simulink model "Longitudinal_Real"  (R2024b)
settings: Solver=VariableStepAuto  StartTime=0.0  StopTime=720  RelTol=1e-3
undefined symbols (not defined in the file): Kd_3, Ki_2, Ki_3, Ki_4, Ki_5, Kp_1, Kp_2, Kp_3, Kp_4, Kp_5
libraries: simulink x18, slpidlib x5
settings Model: Creator=GH-X-ST  LastModifiedBy=GH-X-ST

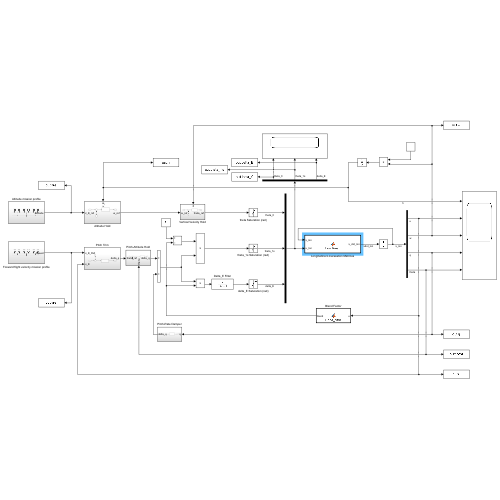
[thumbnail: Simulink's stored preview of the top-level diagram]
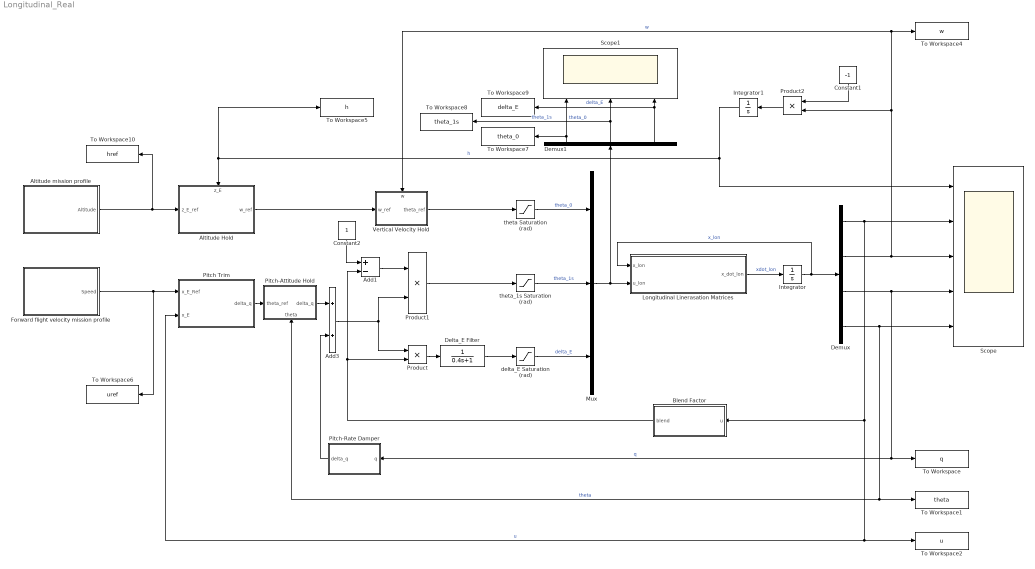
== system Longitudinal_Real ==
  Add1 : Sum  Inputs=+-
  Add3 : Sum
  Altitude Hold : Subsystem
      settings: PortSchema="{\"entries\":[{\"content\":{\"sides\":[{\"content\":{\"connectorIds\":[\"In1\"]},\"type\":\"ConnectorPlacement.EquallySpacedRectSide\",\"uuid\":\"786fe27b-9d32-4a4b-ba58-745251b51298\"},{\"content\":{\"connectorIds\":[\"Out1\"],\"side\":\"RIGHT\"},\"type\":\"ConnectorPlacement.EquallySpacedRectSide\",\"uuid\":\"c3e63844-28f7-4108-b9b9-8f5ae49ef2b7\"},{\"content\":{\"connectorIds\":[\"In2\"],\"side\":\"TOP\"},\"type\":\"ConnectorPlacement.EquallySpacedRectSide\",\"uuid\":\"709e7f88-d3c1-4cf0-9a6f-fe71781ed8e6\"}]},\"type\":\"ConnectorPlacement.EquallySpacedConnector\",\"uuid\":\"916bac8a-d735-4a54-bfae-f4eae304bdce\"}],\"packageUris\":[\"http://schema.mathworks.com/mf0/Connector/R2020b\"],\"version\":\"1.0\"}"
  Altitude mission profile : Subsystem
  Blend Factor : MATLAB Function  TreatAsAtomicUnit=on
  Constant1 : Constant  Value=-1
  Constant2 : Constant
  Delta_E Filter : TransferFcn  Denominator=[0.4 1]
  Demux : Demux
  Demux1 : Demux  Outputs=3
  Forward flight velocity mission profile : Subsystem
  Integrator : Integrator  InitialCondition=[0.000001; 0; 0; 0]
  Integrator1 : Integrator  InitialCondition=135  ContinuousStateAttributes='h'
  Longitudinal Linerasation Matrices : MATLAB Function  TreatAsAtomicUnit=on
  Mux : Mux  Inputs=3
  Pitch Trim : Subsystem
  Pitch-Attitude Hold : Subsystem
      settings: PortSchema="{\"entries\":[{\"content\":{\"sides\":[{\"content\":{\"connectorIds\":[\"In1\"]},\"type\":\"ConnectorPlacement.EquallySpacedRectSide\",\"uuid\":\"6ee333b9-9b69-42fd-975a-4580f9624540\"},{\"content\":{\"connectorIds\":[\"Out1\"],\"side\":\"RIGHT\"},\"type\":\"ConnectorPlacement.EquallySpacedRectSide\",\"uuid\":\"6a43d978-a0a5-4636-bfdb-b097e996a039\"},{\"content\":{\"side\":\"TOP\"},\"type\":\"ConnectorPlacement.EquallySpacedRectSide\",\"uuid\":\"00f937d1-ecc9-42d4-adf8-d8f1b79c75a6\"},{\"content\":{\"connectorIds\":[\"In2\"],\"side\":\"BOTTOM\"},\"type\":\"ConnectorPlacement.EquallySpacedRectSide\",\"uuid\":\"809403f9-594f-4491-8a7d-ee0f8643f57e\"}]},\"type\":\"ConnectorPlacement.EquallySpacedConnector\",\"uuid\":\"362aafbc-ebc0-4bb3-8c4e-be284a8bc83f\"}],\"packageUris\":[\"http://schema.mathworks.com/mf0/Connector/R2020b\"],\"version\":\"1.0\"}"
  Pitch-Rate Damper : Subsystem
  Product : Product
  Product1 : Product
  Product2 : Product
  Scope : Scope  NumInputPorts=5
  Scope1 : Scope  NumInputPorts=3
  To Workspace : ToWorkspace  VariableName=q  SaveFormat=Timeseries  SampleTime=-1
  To Workspace1 : ToWorkspace  VariableName=theta  SaveFormat=Timeseries  SampleTime=-1
  To Workspace10 : ToWorkspace  VariableName=href  SaveFormat=Timeseries  SampleTime=-1
  To Workspace2 : ToWorkspace  VariableName=u  SaveFormat=Timeseries  SampleTime=-1
  To Workspace4 : ToWorkspace  VariableName=w  SaveFormat=Timeseries  SampleTime=-1
  To Workspace5 : ToWorkspace  VariableName=h  SaveFormat=Timeseries  SampleTime=-1
  To Workspace6 : ToWorkspace  VariableName=uref  SaveFormat=Timeseries  SampleTime=-1
  To Workspace7 : ToWorkspace  VariableName=theta_0  SaveFormat=Timeseries  SampleTime=-1
  To Workspace8 : ToWorkspace  VariableName=theta_1s  SaveFormat=Timeseries  SampleTime=-1
  To Workspace9 : ToWorkspace  VariableName=delta_E  SaveFormat=Timeseries  SampleTime=-1
  Vertical Velocity Hold : Subsystem
      settings: PortSchema="{\"entries\":[{\"content\":{\"sides\":[{\"content\":{\"connectorIds\":[\"In1\"]},\"type\":\"ConnectorPlacement.EquallySpacedRectSide\",\"uuid\":\"6ee333b9-9b69-42fd-975a-4580f9624540\"},{\"content\":{\"connectorIds\":[\"Out1\"],\"side\":\"RIGHT\"},\"type\":\"ConnectorPlacement.EquallySpacedRectSide\",\"uuid\":\"6a43d978-a0a5-4636-bfdb-b097e996a039\"},{\"content\":{\"connectorIds\":[\"In2\"],\"side\":\"TOP\"},\"type\":\"ConnectorPlacement.EquallySpacedRectSide\",\"uuid\":\"00f937d1-ecc9-42d4-adf8-d8f1b79c75a6\"},{\"content\":{\"side\":\"BOTTOM\"},\"type\":\"ConnectorPlacement.EquallySpacedRectSide\",\"uuid\":\"64d125d6-056c-4640-9df5-5340aaf5f7d1\"}]},\"type\":\"ConnectorPlacement.EquallySpacedConnector\",\"uuid\":\"362aafbc-ebc0-4bb3-8c4e-be284a8bc83f\"}],\"packageUris\":[\"http://schema.mathworks.com/mf0/Connector/R2020b\"],\"version\":\"1.0\"}"
  delta_E Saturation (rad) : Saturate  UpperLimit=deg2rad(11)  LowerLimit=deg2rad(-11)
  theta Saturation (rad) : Saturate  UpperLimit=deg2rad(+20)  LowerLimit=deg2rad(-6)
  theta_1s Saturation (rad) : Saturate  UpperLimit=deg2rad(6)  LowerLimit=deg2rad(-6)
  wires:
  Longitudinal Linerasation Matrices/1(x_dot_lon) -> Integrator/1  "xdot_lon"
  Integrator/1 -> Longitudinal Linerasation Matrices/1(x_lon), Demux/1  "x_lon"
  Demux/1 -> Scope/2, Blend Factor/1(u), To Workspace2/1, Pitch Trim/2(x_E)  "u"
  Demux/2 -> Vertical Velocity Hold/2(w), To Workspace4/1, Product2/2, Scope/3  "w"
  Demux/3 -> Scope/4, To Workspace/1, Pitch-Rate Damper/1(q)  "q"
  Demux/4 -> Scope/5, To Workspace1/1, Pitch-Attitude Hold/2(theta)  "theta"
  Blend Factor/1(blend) -> Add1/2, Product/2
  Pitch-Attitude Hold/1(delta_q) -> Add3/1
  Constant2/1 -> Add1/1
  Add1/1 -> Product1/1
  Mux/1 -> Demux1/1, Longitudinal Linerasation Matrices/2(u_lon)
  Demux1/3 -> To Workspace9/1, Scope1/3  "delta_E"
  Demux1/2 -> Scope1/2, To Workspace8/1  "theta_1s"
  Demux1/1 -> Scope1/1, To Workspace7/1  "theta_0"
  Product/1 -> Delta_E Filter/1
  Pitch-Rate Damper/1(delta_q) -> Add3/2
  Constant1/1 -> Product2/1
  Product2/1 -> Integrator1/1
  Integrator1/1 -> Scope/1, Altitude Hold/2(z_E), To Workspace5/1  "h"
  Altitude Hold/1(w_ref) -> Vertical Velocity Hold/1(w_ref)
  Add3/1 -> Product1/2, Product/1
  Pitch Trim/1(delta_q) -> Pitch-Attitude Hold/1(theta_ref)
  Delta_E Filter/1 -> delta_E Saturation (rad)/1
  delta_E Saturation (rad)/1 -> Mux/3  "delta_E"
  theta_1s Saturation (rad)/1 -> Mux/2  "theta_1s"
  Product1/1 -> theta_1s Saturation (rad)/1
  Vertical Velocity Hold/1(theta_ref) -> theta Saturation (rad)/1
  theta Saturation (rad)/1 -> Mux/1  "theta_0"
  Altitude mission profile/1(Altitude) -> To Workspace10/1, Altitude Hold/1(z_E_ref)
  Forward flight velocity mission profile/1(Speed) -> To Workspace6/1, Pitch Trim/1(x_E_Ref)

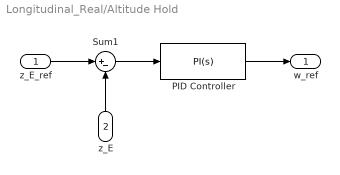
== system Longitudinal_Real/Altitude Hold ==
  z_E_ref : Inport
  z_E : Inport  Port=2
  PID Controller : slpidlib/PID Controller  Controller=PI  Form=Parallel  TimeDomain=Continuous-time  UseExternalTs=off  SampleTime=-1  IntegratorMethod=Forward Euler  FilterMethod=Forward Euler  ControllerParametersSource=internal  P=Kp_5  I=Ki_5  UseKiTs=off  D=0.005  UseExternalDerivativeSource=off  N=100  UseFilter=on  TunerSelectOption=Transfer Function Based (PID Tuner App)  InitialConditionSource=internal  InitialConditionForIntegrator=0  InitialConditionForFilter=0  DifferentiatorICPrevScaledInput=0  ExternalReset=none  TrackingMode=off  Kt=1  LimitOutput=on  SatLimitsSource=internal  UpperSaturationLimit=1  LowerSaturationLimit=-1  LinearizeAsGain=on  AntiWindupMode=none  Kb=1  LimitIntegrator=off  UpperIntegratorSaturationLimit=inf  LowerIntegratorSaturationLimit=-inf  POutMin=[]  POutMax=[]  IOutMin=[]  IOutMax=[]  DOutMin=[]  DOutMax=[]  NOutMin=[]  NOutMax=[]  SumOutMin=[]  SumOutMax=[]  SaturationOutMin=[]  SaturationOutMax=[]  PParamMin=[]  PParamMax=[]  IParamMin=[]  IParamMax=[]  DParamMin=[]  DParamMax=[]  NParamMin=[]  NParamMax=[]  KbParamMin=[]  KbParamMax=[]  KtParamMin=[]  KtParamMax=[]  KbOutMin=[]  KbOutMax=[]  KtOutMin=[]  KtOutMax=[]  IntegratorOutMin=[]  IntegratorOutMax=[]  FilterOutMin=[]  FilterOutMax=[]  SumI1OutMin=[]  SumI1OutMax=[]  SumI2OutMin=[]  SumI2OutMax=[]  SumI3OutMin=[]  SumI3OutMax=[]  SumI4OutMin=[]  SumI4OutMax=[]  SumDOutMin=[]  SumDOutMax=[]  DifferentiatorOutMin=[]  DifferentiatorOutMax=[]  FilterDiffOutCoefMin=[]  FilterDiffOutCoefMax=[]  ReciprocalOutMin=[]  ReciprocalOutMax=[]  SumDenOutMin=[]  SumDenOutMax=[]  SumNumOutMin=[]  SumNumOutMax=[]  DivideOutMin=[]  DivideOutMax=[]  UdiffTsProdOutMin=[]  UdiffTsProdOutMax=[]  NTsProdOutMin=[]  NTsProdOutMax=[]  UintegralTsProdOutMin=[]  UintegralTsProdOutMax=[]  UngainTsProdOutMin=[]  UngainTsProdOutMax=[]  ClampingZeroOutDataTypeStr=Inherit: Inherit via back propagation  ClampingZeroOutMin=[]  ClampingZeroOutMax=[]  FilterDenConstantOutDataTypeStr=Inherit: Inherit via back propagation  FilterDenConstantOutMin=[]  FilterDenConstantOutMax=[]  PCopyOutDataTypeStr=Inherit: Inherit via back propagation  PCopyOutMin=[]  PCopyOutMax=[]  NCopyOutDataTypeStr=Inherit: Inherit via back propagation  NCopyOutMin=[]  NCopyOutMax=[]  IntegratorContinuousStateAttributes=''  IntegratorStateMustResolveToSignalObject=off  IntegratorRTWStateStorageClass=Auto  FilterContinuousStateAttributes=''  FilterStateMustResolveToSignalObject=off  FilterRTWStateStorageClass=Auto  ParallelPVariant=InternalParameters  IdealPVariant=Disabled  IVariant=InternalParameters  DVariant=Disabled  IntegratorVariant=Continuous  SatVariant=Enabled  AWVariant=Passthrough  PCopyVariant=Disabled  TRVariant=Disabled  FdbkBlocksVariant=Forward  IdealPFdbkVariant=Disabled  SatFdbkVariant=Disabled  DerivativeFilterVariant=Disabled  NVariant=Disabled  NCopyVariant=Disabled_SignalSpec  FilterICVariant=Disabled  IntegratorICVariant=InternalICs  ExternalResetVariant=Disabled  TRSumVariant=Passthrough  SumFdbkVariant=Disabled  SumVariant=Sum_PI  TsampFilterVariant=InternalTs  TsampNgainVariant=Passthrough  TsampIntegralVariant=Disabled_SignalSpec  ExternalSaturationOutDataTypeStr=Inherit: Same as second input  DerivativeSourceVariant=Disabled  PreIntVariant=InternalPreInt
  Sum1 : Sum  Inputs=|+-
  w_ref : Outport
  wires:
  PID Controller/1 -> w_ref/1
  Sum1/1 -> PID Controller/1
  z_E_ref/1 -> Sum1/1
  z_E/1 -> Sum1/2

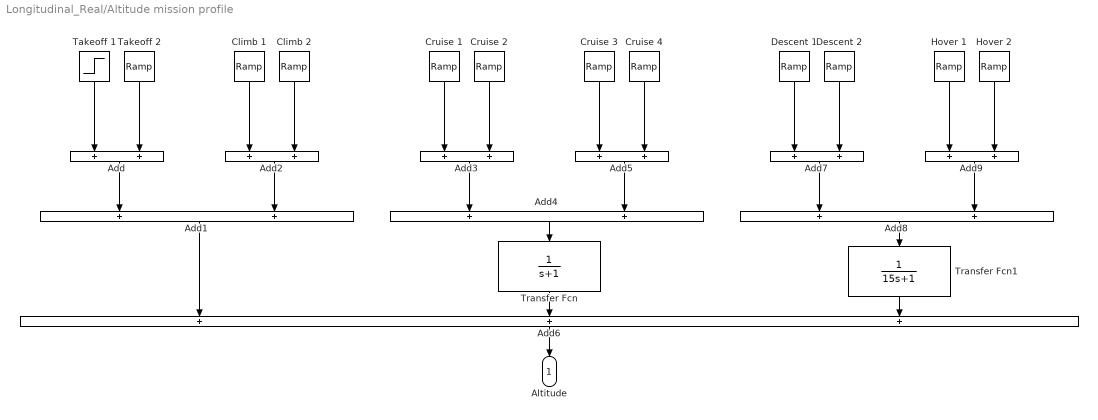
== system Longitudinal_Real/Altitude mission profile ==
  Add{,1..5,7..9} (9 alike) : Sum
  Add6 : Sum  Inputs=+++
  Climb 1 : simulink/Sources/Ramp  slope=0.4  start=50  InitialOutput=0
  Climb 2 : simulink/Sources/Ramp  slope=-0.4  start=100  InitialOutput=0
  Cruise 1 : simulink/Sources/Ramp  slope=0.1  start=100  InitialOutput=0
  Cruise 2 : simulink/Sources/Ramp  slope=-0.1  start=200  InitialOutput=0
  Cruise 3 : simulink/Sources/Ramp  slope=0  start=200  InitialOutput=0
  Cruise 4 : simulink/Sources/Ramp  slope=0  start=350  InitialOutput=0
  Descent 1 : simulink/Sources/Ramp  slope=-12/70  start=350  InitialOutput=0
  Descent 2 : simulink/Sources/Ramp  slope=12/70  start=475  InitialOutput=0
  Hover 1 : simulink/Sources/Ramp  slope=0  start=475  InitialOutput=0
  Hover 2 : simulink/Sources/Ramp  slope=0  start=600  InitialOutput=0
  Takeoff 1 : Step  Time=0  Before=135  After=150  SampleTime=0
  Takeoff 2 : simulink/Sources/Ramp  slope=0  start=50  InitialOutput=0
  Transfer Fcn : TransferFcn  Denominator=[1 1]
  Transfer Fcn1 : TransferFcn  Denominator=[15 1]
  Altitude : Outport
  wires:
  Add1/1 -> Add6/1
  Climb 2/1 -> Add2/2
  Add4/1 -> Transfer Fcn/1
  Climb 1/1 -> Add2/1
  Hover 1/1 -> Add9/1
  Add7/1 -> Add8/1
  Descent 1/1 -> Add7/1
  Add9/1 -> Add8/2
  Hover 2/1 -> Add9/2
  Add8/1 -> Transfer Fcn1/1
  Add2/1 -> Add1/2
  Add3/1 -> Add4/1
  Add5/1 -> Add4/2
  Cruise 2/1 -> Add3/2
  Cruise 4/1 -> Add5/2
  Cruise 1/1 -> Add3/1
  Cruise 3/1 -> Add5/1
  Descent 2/1 -> Add7/2
  Takeoff 2/1 -> Add/2
  Takeoff 1/1 -> Add/1
  Add/1 -> Add1/1
  Add6/1 -> Altitude/1
  Transfer Fcn/1 -> Add6/2
  Transfer Fcn1/1 -> Add6/3

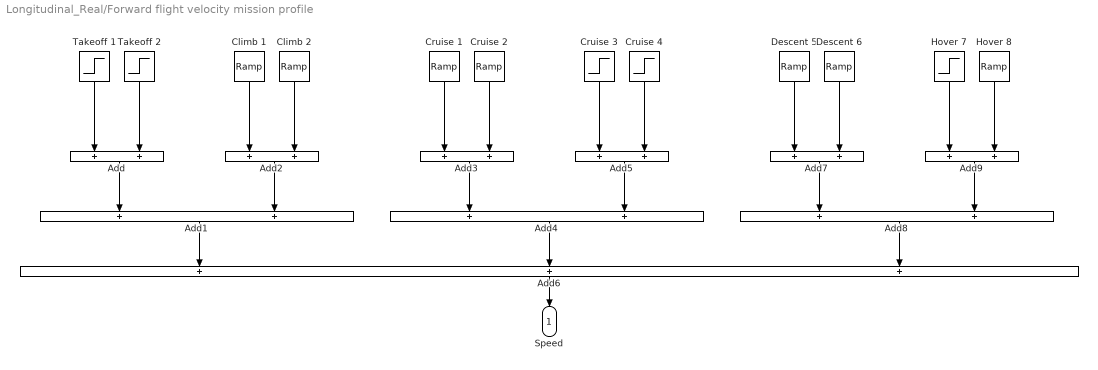
== system Longitudinal_Real/Forward flight velocity mission profile ==
  Add{,1..5,7..9} (9 alike) : Sum
  Add6 : Sum  Inputs=+++
  Climb 1 : simulink/Sources/Ramp  slope=0.4  start=50  InitialOutput=0
  Climb 2 : simulink/Sources/Ramp  slope=-0.4  start=100  InitialOutput=0
  Cruise 1 : simulink/Sources/Ramp  slope=0  start=100  InitialOutput=0
  Cruise 2 : simulink/Sources/Ramp  slope=0  start=200  InitialOutput=0
  Cruise 3 : Step  Time=200  After=22  SampleTime=0
  Cruise 4 : Step  Time=350  After=-37  SampleTime=0
  Descent 5 : simulink/Sources/Ramp  slope=0  start=350  InitialOutput=0
  Descent 6 : simulink/Sources/Ramp  slope=0  start=475  InitialOutput=0
  Hover 7 : Step  Time=475  After=-35  SampleTime=0
  Hover 8 : simulink/Sources/Ramp  slope=0  start=600  InitialOutput=0
  Takeoff 1 : Step  Time=0  After=0  SampleTime=0
  Takeoff 2 : Step  Time=50  After=30  SampleTime=0
  Speed : Outport
  wires:
  Add6/1 -> Speed/1
  Add1/1 -> Add6/1
  Climb 2/1 -> Add2/2
  Add4/1 -> Add6/2
  Climb 1/1 -> Add2/1
  Add7/1 -> Add8/1
  Descent 5/1 -> Add7/1
  Add9/1 -> Add8/2
  Descent 6/1 -> Add7/2
  Hover 8/1 -> Add9/2
  Add8/1 -> Add6/3
  Add2/1 -> Add1/2
  Add3/1 -> Add4/1
  Add5/1 -> Add4/2
  Cruise 1/1 -> Add3/1
  Cruise 4/1 -> Add5/2
  Add/1 -> Add1/1
  Hover 7/1 -> Add9/1
  Takeoff 1/1 -> Add/1
  Takeoff 2/1 -> Add/2
  Cruise 3/1 -> Add5/1
  Cruise 2/1 -> Add3/2

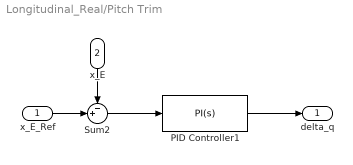
== system Longitudinal_Real/Pitch Trim ==
  x_E_Ref : Inport
  x_E : Inport  Port=2
  PID Controller1 : slpidlib/PID Controller  Controller=PI  Form=Parallel  TimeDomain=Continuous-time  UseExternalTs=off  SampleTime=-1  IntegratorMethod=Forward Euler  FilterMethod=Forward Euler  ControllerParametersSource=internal  P=Kp_3  I=Ki_3  UseKiTs=off  D=Kd_3  UseExternalDerivativeSource=off  N=100  UseFilter=on  TunerSelectOption=Transfer Function Based (PID Tuner App)  InitialConditionSource=internal  InitialConditionForIntegrator=0  InitialConditionForFilter=0  DifferentiatorICPrevScaledInput=0  ExternalReset=none  TrackingMode=off  Kt=1  LimitOutput=on  SatLimitsSource=internal  UpperSaturationLimit=1  LowerSaturationLimit=-1  LinearizeAsGain=on  AntiWindupMode=none  Kb=1  LimitIntegrator=off  UpperIntegratorSaturationLimit=inf  LowerIntegratorSaturationLimit=-inf  POutMin=[]  POutMax=[]  IOutMin=[]  IOutMax=[]  DOutMin=[]  DOutMax=[]  NOutMin=[]  NOutMax=[]  SumOutMin=[]  SumOutMax=[]  SaturationOutMin=[]  SaturationOutMax=[]  PParamMin=[]  PParamMax=[]  IParamMin=[]  IParamMax=[]  DParamMin=[]  DParamMax=[]  NParamMin=[]  NParamMax=[]  KbParamMin=[]  KbParamMax=[]  KtParamMin=[]  KtParamMax=[]  KbOutMin=[]  KbOutMax=[]  KtOutMin=[]  KtOutMax=[]  IntegratorOutMin=[]  IntegratorOutMax=[]  FilterOutMin=[]  FilterOutMax=[]  SumI1OutMin=[]  SumI1OutMax=[]  SumI2OutMin=[]  SumI2OutMax=[]  SumI3OutMin=[]  SumI3OutMax=[]  SumI4OutMin=[]  SumI4OutMax=[]  SumDOutMin=[]  SumDOutMax=[]  DifferentiatorOutMin=[]  DifferentiatorOutMax=[]  FilterDiffOutCoefMin=[]  FilterDiffOutCoefMax=[]  ReciprocalOutMin=[]  ReciprocalOutMax=[]  SumDenOutMin=[]  SumDenOutMax=[]  SumNumOutMin=[]  SumNumOutMax=[]  DivideOutMin=[]  DivideOutMax=[]  UdiffTsProdOutMin=[]  UdiffTsProdOutMax=[]  NTsProdOutMin=[]  NTsProdOutMax=[]  UintegralTsProdOutMin=[]  UintegralTsProdOutMax=[]  UngainTsProdOutMin=[]  UngainTsProdOutMax=[]  ClampingZeroOutDataTypeStr=Inherit: Inherit via back propagation  ClampingZeroOutMin=[]  ClampingZeroOutMax=[]  FilterDenConstantOutDataTypeStr=Inherit: Inherit via back propagation  FilterDenConstantOutMin=[]  FilterDenConstantOutMax=[]  PCopyOutDataTypeStr=Inherit: Inherit via back propagation  PCopyOutMin=[]  PCopyOutMax=[]  NCopyOutDataTypeStr=Inherit: Inherit via back propagation  NCopyOutMin=[]  NCopyOutMax=[]  IntegratorContinuousStateAttributes=''  IntegratorStateMustResolveToSignalObject=off  IntegratorRTWStateStorageClass=Auto  FilterContinuousStateAttributes=''  FilterStateMustResolveToSignalObject=off  FilterRTWStateStorageClass=Auto  ParallelPVariant=InternalParameters  IdealPVariant=Disabled  IVariant=InternalParameters  DVariant=Disabled  IntegratorVariant=Continuous  SatVariant=Enabled  AWVariant=Passthrough  PCopyVariant=Disabled  TRVariant=Disabled  FdbkBlocksVariant=Forward  IdealPFdbkVariant=Disabled  SatFdbkVariant=Disabled  DerivativeFilterVariant=Disabled  NVariant=Disabled  NCopyVariant=Disabled_SignalSpec  FilterICVariant=Disabled  IntegratorICVariant=InternalICs  ExternalResetVariant=Disabled  TRSumVariant=Passthrough  SumFdbkVariant=Disabled  SumVariant=Sum_PI  TsampFilterVariant=InternalTs  TsampNgainVariant=Passthrough  TsampIntegralVariant=Disabled_SignalSpec  ExternalSaturationOutDataTypeStr=Inherit: Same as second input  DerivativeSourceVariant=Disabled  PreIntVariant=InternalPreInt
  Sum2 : Sum  Inputs=-+|
  delta_q : Outport
  wires:
  x_E/1 -> Sum2/1
  x_E_Ref/1 -> Sum2/2
  PID Controller1/1 -> delta_q/1
  Sum2/1 -> PID Controller1/1

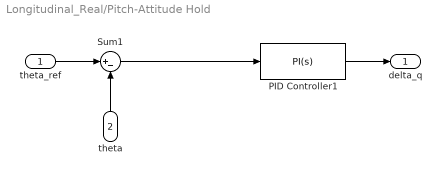
== system Longitudinal_Real/Pitch-Attitude Hold ==
  theta_ref : Inport
  theta : Inport  Port=2
  PID Controller1 : slpidlib/PID Controller  Controller=PI  Form=Parallel  TimeDomain=Continuous-time  UseExternalTs=off  SampleTime=-1  IntegratorMethod=Forward Euler  FilterMethod=Forward Euler  ControllerParametersSource=internal  P=Kp_2  I=Ki_2  UseKiTs=off  D=0.005  UseExternalDerivativeSource=on  N=100  UseFilter=on  TunerSelectOption=Transfer Function Based (PID Tuner App)  InitialConditionSource=internal  InitialConditionForIntegrator=0  InitialConditionForFilter=0  DifferentiatorICPrevScaledInput=0  ExternalReset=none  TrackingMode=off  Kt=1  LimitOutput=on  SatLimitsSource=internal  UpperSaturationLimit=1  LowerSaturationLimit=-1  LinearizeAsGain=on  AntiWindupMode=none  Kb=1  LimitIntegrator=off  UpperIntegratorSaturationLimit=inf  LowerIntegratorSaturationLimit=-inf  POutMin=[]  POutMax=[]  IOutMin=[]  IOutMax=[]  DOutMin=[]  DOutMax=[]  NOutMin=[]  NOutMax=[]  SumOutMin=[]  SumOutMax=[]  SaturationOutMin=[]  SaturationOutMax=[]  PParamMin=[]  PParamMax=[]  IParamMin=[]  IParamMax=[]  DParamMin=[]  DParamMax=[]  NParamMin=[]  NParamMax=[]  KbParamMin=[]  KbParamMax=[]  KtParamMin=[]  KtParamMax=[]  KbOutMin=[]  KbOutMax=[]  KtOutMin=[]  KtOutMax=[]  IntegratorOutMin=[]  IntegratorOutMax=[]  FilterOutMin=[]  FilterOutMax=[]  SumI1OutMin=[]  SumI1OutMax=[]  SumI2OutMin=[]  SumI2OutMax=[]  SumI3OutMin=[]  SumI3OutMax=[]  SumI4OutMin=[]  SumI4OutMax=[]  SumDOutMin=[]  SumDOutMax=[]  DifferentiatorOutMin=[]  DifferentiatorOutMax=[]  FilterDiffOutCoefMin=[]  FilterDiffOutCoefMax=[]  ReciprocalOutMin=[]  ReciprocalOutMax=[]  SumDenOutMin=[]  SumDenOutMax=[]  SumNumOutMin=[]  SumNumOutMax=[]  DivideOutMin=[]  DivideOutMax=[]  UdiffTsProdOutMin=[]  UdiffTsProdOutMax=[]  NTsProdOutMin=[]  NTsProdOutMax=[]  UintegralTsProdOutMin=[]  UintegralTsProdOutMax=[]  UngainTsProdOutMin=[]  UngainTsProdOutMax=[]  ClampingZeroOutDataTypeStr=Inherit: Inherit via back propagation  ClampingZeroOutMin=[]  ClampingZeroOutMax=[]  FilterDenConstantOutDataTypeStr=Inherit: Inherit via back propagation  FilterDenConstantOutMin=[]  FilterDenConstantOutMax=[]  PCopyOutDataTypeStr=Inherit: Inherit via back propagation  PCopyOutMin=[]  PCopyOutMax=[]  NCopyOutDataTypeStr=Inherit: Inherit via back propagation  NCopyOutMin=[]  NCopyOutMax=[]  IntegratorContinuousStateAttributes=''  IntegratorStateMustResolveToSignalObject=off  IntegratorRTWStateStorageClass=Auto  FilterContinuousStateAttributes=''  FilterStateMustResolveToSignalObject=off  FilterRTWStateStorageClass=Auto  ParallelPVariant=InternalParameters  IdealPVariant=Disabled  IVariant=InternalParameters  DVariant=Disabled  IntegratorVariant=Continuous  SatVariant=Enabled  AWVariant=Passthrough  PCopyVariant=Disabled  TRVariant=Disabled  FdbkBlocksVariant=Forward  IdealPFdbkVariant=Disabled  SatFdbkVariant=Disabled  DerivativeFilterVariant=Disabled  NVariant=Passthrough  NCopyVariant=Disabled_SignalSpec  FilterICVariant=Disabled  IntegratorICVariant=InternalICs  ExternalResetVariant=Disabled  TRSumVariant=Passthrough  SumFdbkVariant=Disabled  SumVariant=Sum_PI  TsampFilterVariant=InternalTs  TsampNgainVariant=Passthrough  TsampIntegralVariant=Disabled_SignalSpec  ExternalSaturationOutDataTypeStr=Inherit: Same as second input  DerivativeSourceVariant=Disabled  PreIntVariant=InternalPreInt
  Sum1 : Sum  Inputs=|+-
  delta_q : Outport
  wires:
  PID Controller1/1 -> delta_q/1
  theta_ref/1 -> Sum1/1
  theta/1 -> Sum1/2
  Sum1/1 -> PID Controller1/1

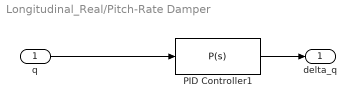
== system Longitudinal_Real/Pitch-Rate Damper ==
  q : Inport
  PID Controller1 : slpidlib/PID Controller  Controller=P  Form=Parallel  TimeDomain=Continuous-time  UseExternalTs=off  SampleTime=-1  IntegratorMethod=Forward Euler  FilterMethod=Forward Euler  ControllerParametersSource=internal  P=Kp_1  I=0.005  UseKiTs=off  D=0.005  UseExternalDerivativeSource=on  N=100  UseFilter=on  TunerSelectOption=Transfer Function Based (PID Tuner App)  InitialConditionSource=internal  InitialConditionForIntegrator=0  InitialConditionForFilter=0  DifferentiatorICPrevScaledInput=0  ExternalReset=none  TrackingMode=off  Kt=1  LimitOutput=on  SatLimitsSource=internal  UpperSaturationLimit=1  LowerSaturationLimit=-1  LinearizeAsGain=on  AntiWindupMode=none  Kb=1  LimitIntegrator=off  UpperIntegratorSaturationLimit=inf  LowerIntegratorSaturationLimit=-inf  POutMin=[]  POutMax=[]  IOutMin=[]  IOutMax=[]  DOutMin=[]  DOutMax=[]  NOutMin=[]  NOutMax=[]  SumOutMin=[]  SumOutMax=[]  SaturationOutMin=[]  SaturationOutMax=[]  PParamMin=[]  PParamMax=[]  IParamMin=[]  IParamMax=[]  DParamMin=[]  DParamMax=[]  NParamMin=[]  NParamMax=[]  KbParamMin=[]  KbParamMax=[]  KtParamMin=[]  KtParamMax=[]  KbOutMin=[]  KbOutMax=[]  KtOutMin=[]  KtOutMax=[]  IntegratorOutMin=[]  IntegratorOutMax=[]  FilterOutMin=[]  FilterOutMax=[]  SumI1OutMin=[]  SumI1OutMax=[]  SumI2OutMin=[]  SumI2OutMax=[]  SumI3OutMin=[]  SumI3OutMax=[]  SumI4OutMin=[]  SumI4OutMax=[]  SumDOutMin=[]  SumDOutMax=[]  DifferentiatorOutMin=[]  DifferentiatorOutMax=[]  FilterDiffOutCoefMin=[]  FilterDiffOutCoefMax=[]  ReciprocalOutMin=[]  ReciprocalOutMax=[]  SumDenOutMin=[]  SumDenOutMax=[]  SumNumOutMin=[]  SumNumOutMax=[]  DivideOutMin=[]  DivideOutMax=[]  UdiffTsProdOutMin=[]  UdiffTsProdOutMax=[]  NTsProdOutMin=[]  NTsProdOutMax=[]  UintegralTsProdOutMin=[]  UintegralTsProdOutMax=[]  UngainTsProdOutMin=[]  UngainTsProdOutMax=[]  ClampingZeroOutDataTypeStr=Inherit: Inherit via back propagation  ClampingZeroOutMin=[]  ClampingZeroOutMax=[]  FilterDenConstantOutDataTypeStr=Inherit: Inherit via back propagation  FilterDenConstantOutMin=[]  FilterDenConstantOutMax=[]  PCopyOutDataTypeStr=Inherit: Inherit via back propagation  PCopyOutMin=[]  PCopyOutMax=[]  NCopyOutDataTypeStr=Inherit: Inherit via back propagation  NCopyOutMin=[]  NCopyOutMax=[]  IntegratorContinuousStateAttributes=''  IntegratorStateMustResolveToSignalObject=off  IntegratorRTWStateStorageClass=Auto  FilterContinuousStateAttributes=''  FilterStateMustResolveToSignalObject=off  FilterRTWStateStorageClass=Auto  ParallelPVariant=InternalParameters  IdealPVariant=Disabled  IVariant=Disabled  DVariant=Disabled  IntegratorVariant=Disabled  SatVariant=Enabled  AWVariant=Disabled  PCopyVariant=Disabled  TRVariant=Disabled  FdbkBlocksVariant=Forward  IdealPFdbkVariant=Disabled  SatFdbkVariant=Disabled  DerivativeFilterVariant=Disabled  NVariant=Passthrough  NCopyVariant=Disabled_SignalSpec  FilterICVariant=Disabled  IntegratorICVariant=Disabled  ExternalResetVariant=Disabled  TRSumVariant=Passthrough  SumFdbkVariant=Disabled  SumVariant=Passthrough_P  TsampFilterVariant=InternalTs  TsampNgainVariant=Passthrough  TsampIntegralVariant=Disabled_SignalSpec  ExternalSaturationOutDataTypeStr=Inherit: Same as second input  DerivativeSourceVariant=Disabled  PreIntVariant=InternalPreInt
  delta_q : Outport
  wires:
  PID Controller1/1 -> delta_q/1
  q/1 -> PID Controller1/1

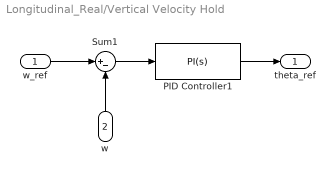
== system Longitudinal_Real/Vertical Velocity Hold ==
  w_ref : Inport
  w : Inport  Port=2
  PID Controller1 : slpidlib/PID Controller  Controller=PI  Form=Parallel  TimeDomain=Continuous-time  UseExternalTs=off  SampleTime=-1  IntegratorMethod=Forward Euler  FilterMethod=Forward Euler  ControllerParametersSource=internal  P=Kp_4  I=Ki_4  UseKiTs=off  D=0.005  UseExternalDerivativeSource=on  N=100  UseFilter=on  TunerSelectOption=Transfer Function Based (PID Tuner App)  InitialConditionSource=internal  InitialConditionForIntegrator=0  InitialConditionForFilter=0  DifferentiatorICPrevScaledInput=0  ExternalReset=none  TrackingMode=off  Kt=1  LimitOutput=on  SatLimitsSource=internal  UpperSaturationLimit=1  LowerSaturationLimit=-1  LinearizeAsGain=on  AntiWindupMode=none  Kb=1  LimitIntegrator=off  UpperIntegratorSaturationLimit=inf  LowerIntegratorSaturationLimit=-inf  POutMin=[]  POutMax=[]  IOutMin=[]  IOutMax=[]  DOutMin=[]  DOutMax=[]  NOutMin=[]  NOutMax=[]  SumOutMin=[]  SumOutMax=[]  SaturationOutMin=[]  SaturationOutMax=[]  PParamMin=[]  PParamMax=[]  IParamMin=[]  IParamMax=[]  DParamMin=[]  DParamMax=[]  NParamMin=[]  NParamMax=[]  KbParamMin=[]  KbParamMax=[]  KtParamMin=[]  KtParamMax=[]  KbOutMin=[]  KbOutMax=[]  KtOutMin=[]  KtOutMax=[]  IntegratorOutMin=[]  IntegratorOutMax=[]  FilterOutMin=[]  FilterOutMax=[]  SumI1OutMin=[]  SumI1OutMax=[]  SumI2OutMin=[]  SumI2OutMax=[]  SumI3OutMin=[]  SumI3OutMax=[]  SumI4OutMin=[]  SumI4OutMax=[]  SumDOutMin=[]  SumDOutMax=[]  DifferentiatorOutMin=[]  DifferentiatorOutMax=[]  FilterDiffOutCoefMin=[]  FilterDiffOutCoefMax=[]  ReciprocalOutMin=[]  ReciprocalOutMax=[]  SumDenOutMin=[]  SumDenOutMax=[]  SumNumOutMin=[]  SumNumOutMax=[]  DivideOutMin=[]  DivideOutMax=[]  UdiffTsProdOutMin=[]  UdiffTsProdOutMax=[]  NTsProdOutMin=[]  NTsProdOutMax=[]  UintegralTsProdOutMin=[]  UintegralTsProdOutMax=[]  UngainTsProdOutMin=[]  UngainTsProdOutMax=[]  ClampingZeroOutDataTypeStr=Inherit: Inherit via back propagation  ClampingZeroOutMin=[]  ClampingZeroOutMax=[]  FilterDenConstantOutDataTypeStr=Inherit: Inherit via back propagation  FilterDenConstantOutMin=[]  FilterDenConstantOutMax=[]  PCopyOutDataTypeStr=Inherit: Inherit via back propagation  PCopyOutMin=[]  PCopyOutMax=[]  NCopyOutDataTypeStr=Inherit: Inherit via back propagation  NCopyOutMin=[]  NCopyOutMax=[]  IntegratorContinuousStateAttributes=''  IntegratorStateMustResolveToSignalObject=off  IntegratorRTWStateStorageClass=Auto  FilterContinuousStateAttributes=''  FilterStateMustResolveToSignalObject=off  FilterRTWStateStorageClass=Auto  ParallelPVariant=InternalParameters  IdealPVariant=Disabled  IVariant=InternalParameters  DVariant=Disabled  IntegratorVariant=Continuous  SatVariant=Enabled  AWVariant=Passthrough  PCopyVariant=Disabled  TRVariant=Disabled  FdbkBlocksVariant=Forward  IdealPFdbkVariant=Disabled  SatFdbkVariant=Disabled  DerivativeFilterVariant=Disabled  NVariant=Passthrough  NCopyVariant=Disabled_SignalSpec  FilterICVariant=Disabled  IntegratorICVariant=InternalICs  ExternalResetVariant=Disabled  TRSumVariant=Passthrough  SumFdbkVariant=Disabled  SumVariant=Sum_PI  TsampFilterVariant=InternalTs  TsampNgainVariant=Passthrough  TsampIntegralVariant=Disabled_SignalSpec  ExternalSaturationOutDataTypeStr=Inherit: Same as second input  DerivativeSourceVariant=Disabled  PreIntVariant=InternalPreInt
  Sum1 : Sum  Inputs=|+-
  theta_ref : Outport
  wires:
  PID Controller1/1 -> theta_ref/1
  Sum1/1 -> PID Controller1/1
  w_ref/1 -> Sum1/1
  w/1 -> Sum1/2

== matlab function Longitudinal_Real/Longitudinal Linerasation Matrices ==
  data: x_lon input; u_lon input; x_dot_lon output
function x_dot_lon = Lon_linear(x_lon, u_lon)
% Author:
%   Hanchen Li (hl3422@ic.ac.uk)
%
% Inputs:
%   x_lon     - [u, w, q, theta]
%   u         - Forward velocity (m/s)
%   w         - Vertical velocity (m/s)
%   q         - Pitch rate (rad/s)
%   theta     - Euler pitch angle (rad)
%
%   u_lon     - [theta_0, theta_1s, delta_E]
%   theta_0   - Average rotor collective (rad)
%   theta_1s  - Longitudinal cyclic (rad)
%   delta_E   - Elevator deflection (rad)
%
% Outputs:
%   x_dot_lon - [u_dot, w_dot, q_dot, theta_dot]

%% 0 Extract Parameters
u     = x_lon(1);
% w     = x_lon(2);
% q     = x_lon(3);
% theta = x_lon(4);

% theta_0 = u_lon(1);
% theta_1s = u_lon(2);
% delta_E = u_lon(3);


A_lon = ...
[-0.00723802383207751	-1.35323092947785e-20	-0.766629187912504	-9.80664998365558;
-3.64153152077051e-10	-0.626783991819480	0	0;
0.000872483038786669	1.53518643043251e-21	0.0942177477514433	0;
0	0	1	0];

B_lon = ...
[-2.41065865317012e-18	-5.17979000748556	0;
-111.654787649114	0	0;
2.95095583193773e-19	0.636589574236795	0;
0	0	0];

%% 3 Output
x_dot_lon = A_lon * x_lon + B_lon * u_lon;

end

== matlab function Longitudinal_Real/Blend Factor ==
  data: blend output; u input
function blend = Blend_pitch(u)
% Author:
%   Hanchen Li (hl3422@ic.ac.uk)
%
% Inputs:
%   u         - Forward velocity (m/s)
%
% Outputs:
%   blend     - blend factor

%% 1 Decide blend factor

if abs(u) < 1e-4

    blend = 0;

elseif abs(u) < 90.3

    blend = u / (90.3 / 0.8);

else

    blend = 0.8;

end

end
